simulink model "ProposedSISOmodeling"  (R2020a)
settings: Solver=VariableStepAuto  StartTime=0.0  StopTime=240000  RelTol=1e-3
undefined symbols (not defined in the file): Kd, Ku
libraries: cstblocks x4
settings Model: Creator=User  LastModifiedBy=User
settings SolverCC: AlgebraicLoopSolver=LineSearch

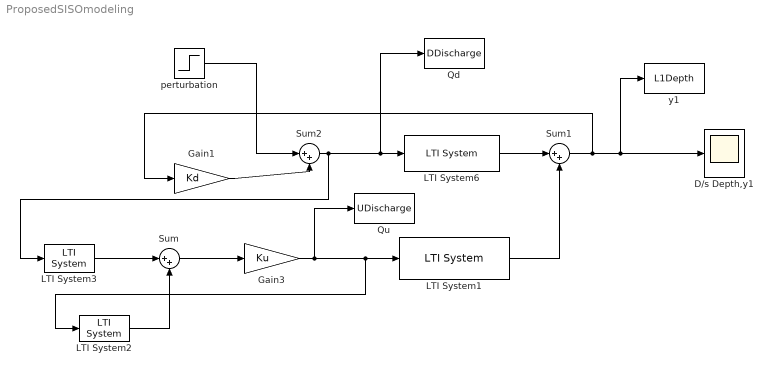
== system ProposedSISOmodeling ==
  D/s Depth,y1 : Scope
  Gain1 : Gain  Gain=Kd
  Gain3 : Gain  Gain=Ku
  LTI System1 : cstblocks/LTI System  sys=P21  IC=[]
  LTI System2 : cstblocks/LTI System  sys=P11  IC=[]
  LTI System3 : cstblocks/LTI System  sys=P12  IC=[]
  LTI System6 : cstblocks/LTI System  sys=P22  IC=[]
  Qd : ToWorkspace  VariableName=DDischarge  SaveFormat=Timeseries  SampleTime=-1
  Qu : ToWorkspace  VariableName=UDischarge  SaveFormat=Timeseries  SampleTime=-1
  Sum : Sum  Inputs=|++
  Sum1 : Sum  Inputs=|++
  Sum2 : Sum  Inputs=|++
  perturbation : Step  Time=1200  After=0.5  SampleTime=0
  y1 : ToWorkspace  VariableName=L1Depth  SaveFormat=Timeseries  SampleTime=-1
  wires:
  Sum1/1 -> Gain1/1, D/s Depth,y1/1, y1/1
  LTI System6/1 -> Sum1/1
  LTI System1/1 -> Sum1/2
  perturbation/1 -> Sum2/1
  Sum2/1 -> Qd/1, LTI System6/1, LTI System3/1
  Gain1/1 -> Sum2/2
  Gain3/1 -> LTI System2/1, LTI System1/1, Qu/1
  Sum/1 -> Gain3/1
  LTI System3/1 -> Sum/1
  LTI System2/1 -> Sum/2
